simulink model "TAYCAN_MODEL"  (R2025b)
settings: Solver=ode23t  StartTime=0.0  StopTime=10000  RelTol=1e-3
values from neighbouring files (symbols this model uses):
  g = 9.81    [DRIVE_CYCLE_GEN.m]    (also in TAYCAN_PARAM_LOAD.m)
  L = 500    [TAYCAN_PARAM_LOAD.m]
  Max_brake_pressure_F_Bar = 200e5    (= 20000000)    [TAYCAN_PARAM_LOAD.m]
  Max_brake_pressure_R_Bar = 200e5    (= 20000000)    [TAYCAN_PARAM_LOAD.m]
  Max_torque_curve_F_Nm = Torque_x * Max_torque_curve_F_set    [Model_Sweeper.m]    (also in TAYCAN_PARAM_LOAD.m = [340;340;340;340;340;340;288.55;247.42;216.63;192.44;173.11;)
  Max_torque_curve_R_Nm = Torque_x * Max_torque_curve_R_set    [Model_Sweeper.m]    (also in TAYCAN_PARAM_LOAD.m = [900.00;900.00;900.00;900.00;900.00;900.00;900.00;898.90;785)
  Max_torque_generator_Nm = -350    [TAYCAN_PARAM_LOAD.m]
  Np = ceil(Ipack / Imax)    [Model_Sweeper.m]    (also in TAYCAN_PARAM_LOAD.m = 33)
  Ns = 198    [TAYCAN_PARAM_LOAD.m]
  regen_bias = 0.3    [TAYCAN_PARAM_LOAD.m]
  RPM_curve_RPM_F = (0:1000:RPM_max_RPM_F)'    [TAYCAN_PARAM_LOAD.m]
  RPM_curve_RPM_R = (0:1000:RPM_max_RPM_R)'    [TAYCAN_PARAM_LOAD.m]
  shift_down_v = shift_down_v_set(ids)    [Model_Sweeper.m]    (also in TAYCAN_PARAM_LOAD.m = 60)
  shift_up_v = shift_up_v_set(ids)    [Model_Sweeper.m]    (also in TAYCAN_PARAM_LOAD.m = 80)
  Tot_vehicle_mass_kg = Vehicle_mass_unladen_kg + Driver_mass_kg + batt_mass    [Model_Sweeper.m]    (also in TAYCAN_PARAM_LOAD.m = 2462.38)
  V_init = 4.2    [TAYCAN_PARAM_LOAD.m]
  VelDist = struct()    [DRIVE_CYCLE_GEN.m]    (also in VelocityVsDistance.mat = )
undefined symbols (not defined in the file or in its folder): Driver_Ki, Driver_Kp, Max_torque_motor_F__Nm, Max_torque_motor_R__Nm, Neg, Pos
libraries: fl_lib x23, nesl_utility x16, sdl_lib x15, batteryecm_lib x1, autolibshared x1
(part 1 of 2)
settings Model: Creator=User  LastModifiedBy=User

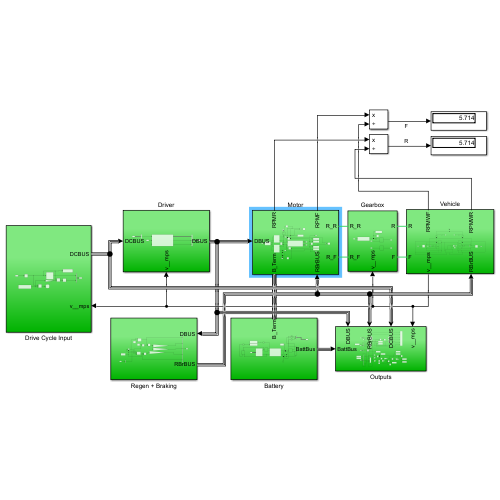
[thumbnail: Simulink's stored preview of the top-level diagram]
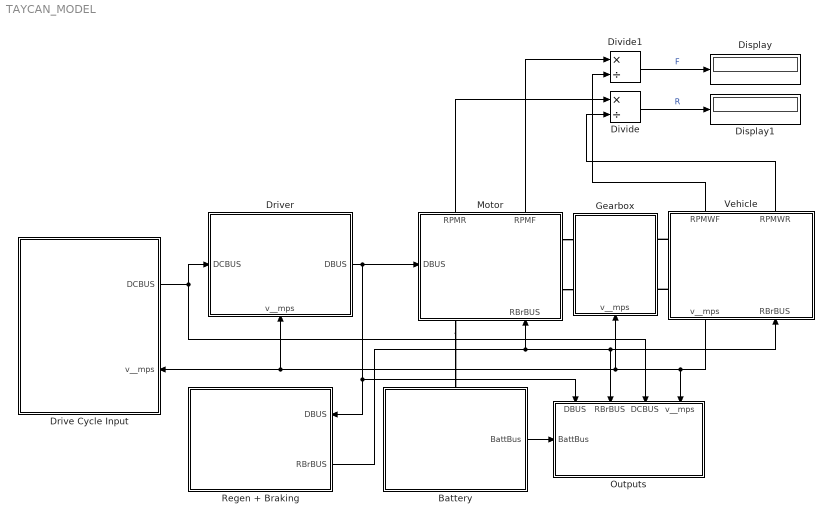
== system TAYCAN_MODEL ==
  Battery : Subsystem
      settings: PortSchema="{\"entries\":[{\"content\":{\"sides\":[{\"content\":{},\"type\":\"ConnectorPlacement.EquallySpacedRectSide\",\"uuid\":\"d14577cf-04a7-401a-8516-23c16a1412d1\"},{\"content\":{\"connectorIds\":[\"Out1\"],\"side\":\"RIGHT\"},\"type\":\"ConnectorPlacement.EquallySpacedRectSide\",\"uuid\":\"4e7522c9-8180-4e2e-bebe-28528e500786\"},{\"content\":{\"connectorIds\":[\"LConn1\"],\"side\":\"TOP\"},\"type\":\"ConnectorPlacement.EquallySpacedRectSide\",\"uuid\":\"3070fdfd-0295-4330-8a72-ca6da87c971c\"}]},\"type\":\"ConnectorPlacement.EquallySpacedConnector\",\"uuid\":\"084f7575-2e43-4328-abba-c452195d4f2d\"}],\"packageUris\":[\"http://schema.mathworks.com/mf0/Connector/R2020b\"],\"version\":\"1.0\"}"
  Display : Display
  Display1 : Display
  Divide : Product  Inputs=*/
  Divide1 : Product  Inputs=*/
  Drive Cycle Input : Subsystem
      settings: PortSchema="{\"entries\":[{\"content\":{\"sides\":[{\"content\":{},\"type\":\"ConnectorPlacement.EquallySpacedRectSide\",\"uuid\":\"0e92d9b4-4c78-4478-9d26-ea78bebdd29e\"},{\"content\":{\"connectorIds\":[\"Out1\",\"In1\"],\"side\":\"RIGHT\"},\"type\":\"ConnectorPlacement.EquallySpacedRectSide\",\"uuid\":\"045dcab9-f8e3-4899-a832-b3da2cc9584c\"},{\"content\":{\"side\":\"TOP\"},\"type\":\"ConnectorPlacement.EquallySpacedRectSide\",\"uuid\":\"84c167e0-eb64-4122-830b-befac4af6cd8\"}]},\"type\":\"ConnectorPlacement.EquallySpacedConnector\",\"uuid\":\"e4b995ab-b6cb-45a0-892e-35ade84b02de\"}],\"packageUris\":[\"http://schema.mathworks.com/mf0/Connector/R2020b\"],\"version\":\"1.0\"}"
  Driver : Subsystem
      settings: PortSchema="{\"entries\":[{\"content\":{\"sides\":[{\"content\":{\"connectorIds\":[\"In1\"]},\"type\":\"ConnectorPlacement.EquallySpacedRectSide\",\"uuid\":\"d14577cf-04a7-401a-8516-23c16a1412d1\"},{\"content\":{\"connectorIds\":[\"Out1\"],\"side\":\"RIGHT\"},\"type\":\"ConnectorPlacement.EquallySpacedRectSide\",\"uuid\":\"4e7522c9-8180-4e2e-bebe-28528e500786\"},{\"content\":{\"side\":\"TOP\"},\"type\":\"ConnectorPlacement.EquallySpacedRectSide\",\"uuid\":\"3070fdfd-0295-4330-8a72-ca6da87c971c\"},{\"content\":{\"connectorIds\":[\"In2\"],\"side\":\"BOTTOM\"},\"type\":\"ConnectorPlacement.EquallySpacedRectSide\",\"uuid\":\"fab3bc93-710b-429a-bed2-c063f5086687\"}]},\"type\":\"ConnectorPlacement.EquallySpacedConnector\",\"uuid\":\"084f7575-2e43-4328-abba-c452195d4f2d\"}],\"packageUris\":[\"http://schema.mathworks.com/mf0/Connector/R2020b\"],\"version\":\"1.0\"}"
  Gearbox : Subsystem
      settings: PortSchema="{\"entries\":[{\"content\":{\"sides\":[{\"content\":{\"connectorIds\":[\"LConn1\",\"LConn2\"]},\"type\":\"ConnectorPlacement.EquallySpacedRectSide\",\"uuid\":\"2cd79867-e1b6-4457-a4ee-a2c785994971\"},{\"content\":{\"connectorIds\":[\"RConn1\",\"RConn2\"],\"side\":\"RIGHT\"},\"type\":\"ConnectorPlacement.EquallySpacedRectSide\",\"uuid\":\"6eaf45d6-e5e8-4926-a6cd-7ecafda04af6\"},{\"content\":{\"side\":\"TOP\"},\"type\":\"ConnectorPlacement.EquallySpacedRectSide\",\"uuid\":\"07ebaeb6-dff9-4024-8855-2c554193f291\"},{\"content\":{\"connectorIds\":[\"In1\"],\"side\":\"BOTTOM\"},\"type\":\"ConnectorPlacement.EquallySpacedRectSide\",\"uuid\":\"50a107d2-832e-4284-8017-5113a03ebe7e\"}]},\"type\":\"ConnectorPlacement.EquallySpacedConnector\",\"uuid\":\"a35e96de-fd7f-4562-8d12-582ef1b75d5a\"}],\"packageUris\":[\"http://schema.mathworks.com/mf0/Connector/R2020b\"],\"version\":\"1.0\"}"
  Motor : Subsystem
      settings: PortSchema="{\"entries\":[{\"content\":{\"sides\":[{\"content\":{\"connectorIds\":[\"In1\"]},\"type\":\"ConnectorPlacement.EquallySpacedRectSide\",\"uuid\":\"4b804e5c-215d-420c-8cbc-4aec0c1bc9ed\"},{\"content\":{\"connectorIds\":[\"RConn1\",\"RConn2\"],\"side\":\"RIGHT\"},\"type\":\"ConnectorPlacement.EquallySpacedRectSide\",\"uuid\":\"7b3b7faa-3322-4a2b-ad45-f514a2b82e50\"},{\"content\":{\"connectorIds\":[\"Out1\",\"Out2\"],\"side\":\"TOP\"},\"type\":\"ConnectorPlacement.EquallySpacedRectSide\",\"uuid\":\"5f544e79-0644-465e-82e8-8009d644c481\"},{\"content\":{\"connectorIds\":[\"RConn3\",\"In2\"],\"side\":\"BOTTOM\"},\"type\":\"ConnectorPlacement.EquallySpacedRectSide\",\"uuid\":\"86807711-4ed8-4d7d-bac7-3eec1d423299\"}]},\"type\":\"ConnectorPlacement.EquallySpacedConnector\",\"uuid\":\"43c8d4a0-f993-46a1-82cf-86d7211b01ab\"}],\"packageUris\":[\"http://schema.mathworks.com/mf0/Connector/R2020b\"],\"version\":\"1.0\"}"
  Outputs : Subsystem
      settings: PortSchema="{\"entries\":[{\"content\":{\"sides\":[{\"content\":{\"connectorIds\":[\"In1\"]},\"type\":\"ConnectorPlacement.EquallySpacedRectSide\",\"uuid\":\"4d7fb8f9-77c0-425d-b0db-40d5e7c47a92\"},{\"content\":{\"side\":\"RIGHT\"},\"type\":\"ConnectorPlacement.EquallySpacedRectSide\",\"uuid\":\"49f936f9-7703-4fe0-b084-ec330908125c\"},{\"content\":{\"connectorIds\":[\"In2\",\"In3\",\"In4\",\"In5\"],\"side\":\"TOP\"},\"type\":\"ConnectorPlacement.EquallySpacedRectSide\",\"uuid\":\"def830fe-aace-4bb5-b5d5-c0664cb17e7e\"}]},\"type\":\"ConnectorPlacement.EquallySpacedConnector\",\"uuid\":\"0cef2ee5-170a-4149-8339-c8d04dee8bf4\"}],\"packageUris\":[\"http://schema.mathworks.com/mf0/Connector/R2020b\"],\"version\":\"1.0\"}"
  Regen + Braking : Subsystem
      settings: PortSchema="{\"entries\":[{\"content\":{\"sides\":[{\"content\":{},\"type\":\"ConnectorPlacement.EquallySpacedRectSide\",\"uuid\":\"79700970-756d-4ec6-8397-66d283bd30cc\"},{\"content\":{\"connectorIds\":[\"In1\",\"Out1\"],\"side\":\"RIGHT\"},\"type\":\"ConnectorPlacement.EquallySpacedRectSide\",\"uuid\":\"0add4294-302d-47bb-9f16-d681ae85b118\"},{\"content\":{\"side\":\"TOP\"},\"type\":\"ConnectorPlacement.EquallySpacedRectSide\",\"uuid\":\"37b62eba-8f15-40cb-afea-bce2353388c7\"}]},\"type\":\"ConnectorPlacement.EquallySpacedConnector\",\"uuid\":\"23d4a446-c033-44e5-854e-98cdd3b391c4\"}],\"packageUris\":[\"http://schema.mathworks.com/mf0/Connector/R2020b\"],\"version\":\"1.0\"}"
  Vehicle : Subsystem
      settings: PortSchema="{\"entries\":[{\"content\":{\"sides\":[{\"content\":{\"connectorIds\":[\"LConn1\",\"LConn2\"]},\"type\":\"ConnectorPlacement.EquallySpacedRectSide\",\"uuid\":\"2204119d-64df-494d-bdf6-dd5790b6a648\"},{\"content\":{\"side\":\"RIGHT\"},\"type\":\"ConnectorPlacement.EquallySpacedRectSide\",\"uuid\":\"957baec1-6ccf-49eb-9229-dff958c69421\"},{\"content\":{\"connectorIds\":[\"Out2\",\"Out3\"],\"side\":\"TOP\"},\"type\":\"ConnectorPlacement.EquallySpacedRectSide\",\"uuid\":\"91f4ac47-3518-4f09-ad19-4e7ac2e2af90\"},{\"content\":{\"connectorIds\":[\"Out1\",\"In1\"],\"side\":\"BOTTOM\"},\"type\":\"ConnectorPlacement.EquallySpacedRectSide\",\"uuid\":\"9fc835d4-3802-4793-8215-dc50523f1a5f\"}]},\"type\":\"ConnectorPlacement.EquallySpacedConnector\",\"uuid\":\"d2ba5914-f28e-4439-8569-04c9912b493f\"}],\"packageUris\":[\"http://schema.mathworks.com/mf0/Connector/R2020b\"],\"version\":\"1.0\"}"
  wires:
  Drive Cycle Input/1(DCBUS) -> Driver/1(DCBUS), Outputs/4(DCBUS)
  Vehicle/1(v__mps) -> Drive Cycle Input/1(v__mps), Driver/2(v__mps), Gearbox/1(v__mps), Outputs/5(v__mps)
  Driver/1(DBUS) -> Outputs/2(DBUS), Regen + Braking/1(DBUS), Motor/1(DBUS)
  Regen + Braking/1(RBrBUS) -> Vehicle/1(RBrBUS), Outputs/3(RBrBUS), Motor/2(RBrBUS)
  Battery/1(BattBus) -> Outputs/1(BattBus)
  Motor/1(RPMR) -> Divide/1
  Vehicle/3(RPMWR) -> Divide/2
  Vehicle/2(RPMWF) -> Divide1/2
  Motor/2(RPMF) -> Divide1/1
  Divide1/1 -> Display/1  "F"
  Divide/1 -> Display1/1  "R"
  connections:
  Motor/RConn3 -- Battery/LConn1
  Motor/RConn1 -- Gearbox/LConn1
  Motor/RConn2 -- Gearbox/LConn2
  Vehicle/LConn1 -- Gearbox/RConn1
  Vehicle/LConn2 -- Gearbox/RConn2

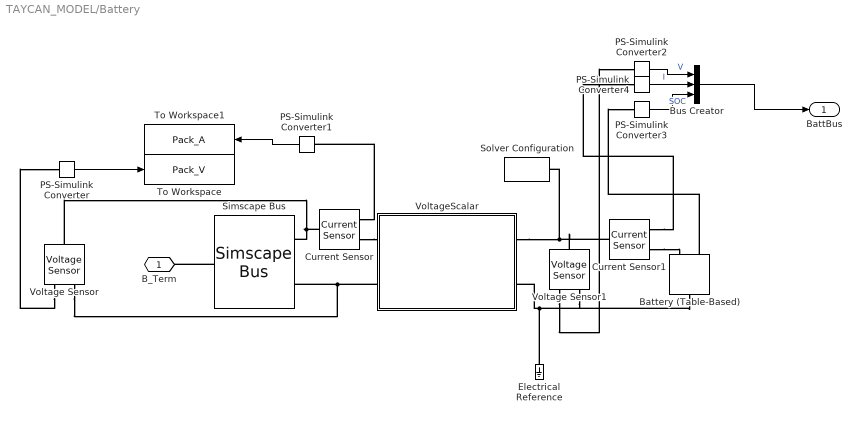
== system TAYCAN_MODEL/Battery ==
  Battery (Table-Based) : batteryecm_lib/Battery (Table-Based)  PartSpecification="{\"CollectionId\":\"SimscapeBatteryShared\",\"CollectionVersion\":\"1.0.0\",\"DatasetId\":\"Molicel|INR_21700_P45B|simscape.battery.batteryTableBased\",\"DisplayName\":\"Molicel:INR_21700_P45B\"}"  SOC_vec=[0 0.01 0.02 0.03 0.04 0.05 0.06 0.07 0.08 0.09 0.1 0.11 0.12 0.13 0.14 0.15 0.16 0.17 0.18 0.19 0.2 0.21 0.22 0.23 0.24 0.25 0.26 0.27 0.28 0.29 0.3 0.31 0.32 0.33 0.34 0.35 0.36 0.37 0.38 0.39 0.4 0.41 0.42 0.43 0.44 0.45 0.46 0.47 0.48 0.49 0.5 0.51 0.52 0.53 0.54 0.55 0.56 0.57 0.58 0.59 0.6 0.61 0.62 0.63 0.64 0.65 0.66 0.67 0.68 0.69 0.7 0.71 0.72 0.73 0.74 0.75 0.76 0.77 0.78 0.79 0.8 0.81 0.82 0.83 0.84 0.85 0.86 0.87 0.88 0.89 0.9 0.91 0.92 0.93 0.94 0.95 0.96 0.97 0.98 0.99 1] % Datasheet derived  T_dependence=simscape.enum.tablebattery.temperature_dependence.yes  prm_dir=simscape.enum.tablebattery.prm_dir.noCurrentDirectionality  T_vec=[-40 -30 -20 0 23 45 60] % Datasheet derived degC  V0_mat=[3.17242 3.17242 3.17242 3.17242 3.17242 3.17242 3.17242;3.18272 3.18272 3.18272 3.18272 3.18272 3.18272 3.18272;3.19302 3.19302 3.19302 3.19302 3.19302 3.19302 3.19302;3.20331 3.20331 3.20331 3.20331 3.20331 3.20331 3.20331;3.21361 3.21361 3.21361 3.21361 3.21361 3.21361 3.21361;3.22391 3.22391 3.22391 3.22391 3.22391 3.22391 3.22391;3.23421 3.23421 3.23421 3.23421 3.23421 3.23421 3.23421;3.24451 3.24451 3.24451 3.24451 3.24451 3.24451 3.24451;3.25481 3.25481 3.25481 3.25481 3.25481 3.25481 3.25481;3.2651 3.2651 3.2651 3.2651 3.2651 3.2651 3.2651;3.2754 3.2754 3.2754 3.2754 3.2754 3.2754 3.2754;3.2857 3.2857 3.2857 3.2857 3.2857 3.2857 3.2857;3.296 3.296 3.296 3.296 3.296 3.296 3.296;3.3063 3.3063 3.3063 3.3063 3.3063 3.3063 3.3063;3.31659 3.31659 3.31659 3.31659 3.31659 3.31659 3.31659;3.32689 3.32689 3.32689 3.32689 3.32689 3.32689 3.32689;3.33719 3.33719 3.33719 3.33719 3.33719 3.33719 3.33719;3.34749 3.34749 3.34749 3.34749 3.34749 3.34749 3.34749;3.35779 3.35779 3.35779 3.35779 3.35779 3.35779 3.35779;3.36809 3.36809 3.36809 3.36809 3.36809 3.36809 3.36809;3.37838 3.37838 3.37838 3.37838 3.37838 3.37838 3.37838;3.38868 3.38868 3.38868 3.38868 3.38868 3.38868 3.38868;3.39898 3.39898 3.39898 3.39898 3.39898 3.39898 3.39898;3.40928 3.40928 3.40928 3.40928 3.40928 3.40928 3.40928;3.41958 3.41958 3.41958 3.41958 3.41958 3.41958 3.41958;3.42988 3.42988 3.42988 3.42988 3.42988 3.42988 3.42988;3.44017 3.44017 3.44017 3.44017 3.44017 3.44017 3.44017;3.45047 3.45047 3.45047 3.45047 3.45047 3.45047 3.45047;3.46077 3.46077 3.46077 3.46077 3.46077 3.46077 3.46077;3.47107 3.47107 3.47107 3.47107 3.47107 3.47107 3.47107;3.48137 3.48137 3.48137 3.48137 3.48137 3.48137 3.48137;3.49166 3.49166 3.49166 3.49166 3.49166 3.49166 3.49166;3.50196 3.50196 3.50196 3.50196 3.50196 3.50196 3.50196;3.51226 3.51226 3.51226 3.51226 3.51226 3.51226 3.51226;3.52256 3.52256 3.52256 3.52256 3.52256 3.52256 3.52256;3.53286 3.53286 3.53286 3.53286 3.53286 3.53286 3.53286;3.54316 3.54316 3.54316 3.54316 3.54316 3.54316 3.54316;3.55345 3.55345 3.55345 3.55345 3.55345 3.55345 3.55345;3.56375 3.56375 3.56375 3.56375 3.56375 3.56375 3.56375;3.57405 3.57405 3.57405 3.57405 3.57405 3.57405 3.57405;3.58435 3.58435 3.58435 3.58435 3.58435 3.58435 3.58435;3.59465 3.59465 3.59465 3.59465 3.59465 3.59465 3.59465;3.60495 3.60495 3.60495 3.60495 3.60495 3.60495 3.60495;3.61524 3.61524 3.61524 3.61524 3.61524 3.61524 3.61524;3.62554 3.62554 3.62554 3.62554 3.62554 3.62554 3.62554;3.63584 3.63584 3.63584 3.63584 3.63584 3.63584 3.63584;3.64614 3.64614 3.64614 3.64614 3.64614 3.64614 3.64614;3.65644 3.65644 3.65644 3.65644 3.65644 3.65644 3.65644;3.66673 3.66673 3.66673 3.66673 3.66673 3.66673 3.66673;3.67703 3.67703 3.67703 3.67703 3.67703 3.67703 3.67703;3.68733 3.68733 3.68733 3.68733 3.68733 3.68733 3.68733;3.69763 3.69763 3.69763 3.69763 3.69763 3.69763 3.69763;3.71041 3.71041 3.71041 3.71041 3.71041 3.71041 3.71041;3.72113 3.72113 3.72113 3.72113 3.72113 3.72113 3.72113;3.72997 3.72997 3.72997 3.72997 3.72997 3.72997 3.72997;3.73882 3.73882 3.73882 3.73882 3.73882 3.73882 3.73882;3.74912 3.74912 3.74912 3.74912 3.74912 3.74912 3.74912;3.75936 3.75936 3.75936 3.75936 3.75936 3.75936 3.75936;3.76951 3.76951 3.76951 3.76951 3.76951 3.76951 3.76951;3.7791 3.7791 3.7791 3.7791 3.7791 3.7791 3.7791;3.78865 3.78865 3.78865 3.78865 3.78865 3.78865 3.78865;3.79787 3.79787 3.79787 3.79787 3.79787 3.79787 3.79787;3.80709 3.80709 3.80709 3.80709 3.80709 3.80709 3.80709;3.8161 3.8161 3.8161 3.8161 3.8161 3.8161 3.8161;3.82509 3.82509 3.82509 3.82509 3.82509 3.82509 3.82509;3.83409 3.83409 3.83409 3.83409 3.83409 3.83409 3.83409;3.84308 3.84308 3.84308 3.84308 3.84308 3.84308 3.84308;3.85207 3.85207 3.85207 3.85207 3.85207 3.85207 3.85207;3.86107 3.86107 3.86107 3.86107 3.86107 3.86107 3.86107;3.87006 3.87006 3.87006 3.87006 3.87006 3.87006 3.87006;3.87901 3.87901 3.87901 3.87901 3.87901 3.87901 3.87901;3.88831 3.88831 3.88831 3.88831 3.88831 3.88831 3.88831;3.89824 3.89824 ...(+1594 chars)] % Datasheet derived V  V0_vec=[3.17242 3.18272 3.19302 3.20331 3.21361 3.22391 3.23421 3.24451 3.25481 3.2651 3.2754 3.2857 3.296 3.3063 3.31659 3.32689 3.33719 3.34749 3.35779 3.36809 3.37838 3.38868 3.39898 3.40928 3.41958 3.42988 3.44017 3.45047 3.46077 3.47107 3.48137 3.49166 3.50196 3.51226 3.52256 3.53286 3.54316 3.55345 3.56375 3.57405 3.58435 3.59465 3.60495 3.61524 3.62554 3.63584 3.64614 3.65644 3.66673 3.67703 3.68733 3.69763 3.71041 3.72113 3.72997 3.73882 3.74912 3.75936 3.76951 3.7791 3.78865 3.79787 3.80709 3.8161 3.82509 3.83409 3.84308 3.85207 3.86107 3.87006 3.87901 3.88831 3.89824 3.90887 3.91951 3.93012 3.94073 3.95138 3.96184 3.97226 3.98268 3.99311 4.0032 4.01221 4.01944 4.02668 4.03286 4.03874 4.04383 4.0488 4.05377 4.05873 4.06312 4.06753 4.07333 4.08117 4.08904 4.09911 4.11111 4.13802 4.16831] % Datasheet derived V  V_range=[2.25 Inf] % Datasheet derived V  R0_mat=[0.3026 0.35142 0.34349 0.24415 0.02095 0.15874 0.14729;0.2941 0.33555 0.32379 0.22614 0.01921 0.13363 0.12249;0.28559 0.31969 0.30408 0.20813 0.01774 0.10853 0.10276;0.27709 0.30382 0.28438 0.19012 0.0166 0.09423 0.0861;0.26858 0.28796 0.26468 0.17211 0.01557 0.07998 0.0748;0.26008 0.27209 0.24498 0.1541 0.01469 0.07024 0.06679;0.25157 0.25623 0.22527 0.1361 0.01398 0.06387 0.05877;0.24307 0.24036 0.20557 0.11861 0.01338 0.0575 0.05275;0.23456 0.2245 0.18587 0.10674 0.01283 0.05113 0.04899;0.22606 0.20863 0.16617 0.09525 0.01239 0.04679 0.04522;0.21755 0.19277 0.14651 0.08799 0.01196 0.0439 0.04145;0.20905 0.1769 0.13098 0.08073 0.01155 0.04101 0.03817;0.20054 0.16103 0.11905 0.07347 0.01116 0.03813 0.03522;0.19204 0.14769 0.11102 0.06895 0.01079 0.03524 0.03228;0.18353 0.13913 0.10517 0.06499 0.01042 0.03235 0.02934;0.17503 0.13157 0.09933 0.06104 0.01007 0.02946 0.0264;0.16653 0.1271 0.09371 0.05708 0.00974 0.02657 0.02345;0.15804 0.12264 0.09094 0.05312 0.00949 0.02417 0.02125;0.15354 0.11817 0.08816 0.04917 0.00924 0.02286 0.01972;0.14976 0.11385 0.08539 0.04748 0.009 0.02156 0.0182;0.14598 0.11213 0.08261 0.04617 0.00876 0.02025 0.01667;0.14219 0.11042 0.08103 0.04487 0.00855 0.01894 0.01515;0.14033 0.10871 0.08035 0.04356 0.00843 0.01763 0.01363;0.13876 0.10699 0.07967 0.04225 0.00832 0.01632 0.0121;0.13718 0.10528 0.07899 0.04094 0.00826 0.01501 0.01058;0.13561 0.10357 0.07831 0.03964 0.00825 0.0137 0.00906;0.13404 0.10198 0.07763 0.03833 0.00825 0.01239 0.00753;0.13247 0.10119 0.07695 0.03702 0.00826 0.01108 0.0065;0.13096 0.10039 0.07627 0.03624 0.00827 0.00977 0.00633;0.13043 0.0996 0.07559 0.03615 0.00828 0.00846 0.00617;0.1299 0.0988 0.07491 0.03606 0.0083 0.00774 0.006;0.12937 0.09801 0.07423 0.03597 0.00834 0.00779 0.00583;0.12883 0.09721 0.07355 0.03588 0.00838 0.00783 0.00567;0.1283 0.09642 0.07301 0.03579 0.00842 0.00787 0.0055;0.12777 0.09585 0.07296 0.0357 0.00848 0.00792 0.00534;0.12724 0.09584 0.07291 0.03561 0.00855 0.00796 0.00517;0.12675 0.09584 0.07286 0.03552 0.00863 0.00801 0.005;0.12643 0.09583 0.0728 0.03543 0.00871 0.00805 0.00484;0.12611 0.09582 0.07275 0.03534 0.00879 0.00809 0.00467;0.12579 0.09582 0.0727 0.03525 0.00887 0.00814 0.0045;0.12547 0.09581 0.07264 0.03526 0.00895 0.00818 0.00434;0.12514 0.0958 0.07259 0.03537 0.00903 0.00823 0.00405;0.12482 0.09579 0.07254 0.03547 0.00911 0.00804 0.00366;0.1245 0.09579 0.07248 0.03558 0.00918 0.00776 0.00327;0.12418 0.09578 0.07243 0.03568 0.00925 0.00748 0.00287;0.12386 0.09577 0.07231 0.03579 0.00931 0.0072 0.00248;0.12354 0.09576 0.0721 0.03589 0.00938 0.00692 0.00209;0.12322 0.09576 0.07189 0.036 0.00946 0.00664 0.0017;0.12301 0.09575 0.07168 0.03611 0.00953 0.00636 0.00131;0.12309 0.09574 0.07147 0.03621 0.00961 0.00608 0.00092;0.12318 0.09573 0.07125 0.0363 0.00968 0.0058 0.00053;0.12326 0.09573 0.07104 0.03637 0.00976 0.00552 0.00014;0.12389 0.09628 0.07138 0.03699 0.00991 0.00579 0.0003;0.12407 0.09637 0.07126 0.03715 0.01 0.0056 0.0003;0.12383 0.09605 0.07073 0.0369 0.01003 0.00504 0.0003;0.12359 0.09573 0.07019 0.03664 0.01006 0.00503 0.0003;0.12367 0.09573 0.06998 0.03671 0.01013 0.00534 0.00063;0.12375 0.09572 0.06975 0.03677 0.01022 0.00564 0.00094;0.1238 0.09569 0.07006 0.0368 0.0103 0.00593 0.00123;0.12372 0.09554 0.07026 0.03671 0.01037 0.00608 0.00139;0.12364 0.09537 0.07046 0.03661 0.01043 0.00623 0.00155;0.12348 0.09514 0.07058 0.03644 0.01049 0.0063 0.00163;0.12333 0.0949 0.07071 0.03627 0.01055 0.00638 0.00171;0.12312 0.09461 0.07078 0.03605 0.01061 0.00641 0.00175;0.12291 0.09433 0.07085 0.03583 0.01066 0.00643 0.00168;0.12271 0.09404 0.07093 0.03568 0.01072 0.00646 0.00161;0.12275 0.09398 0.071 0.03622 0.01077 0.00646 0.00153;0.12316 0.09449 0.07107 0.03677 0.01082 0.00636 0.00145;0.12357 0.095 0.07115 0.03731 0.01088 0.00625 0.00137;0.12398 0.09551 0.07151 0.03785 0.01093 0.00614 0.00129;0.12438 0.09601 0.07221 0.03839 0.01099 0.00602 0.0012;0.12486 0.09659 0.07299 0.039 0.01105 0.00599 0.00119;0.12548 0.09731 0.07391 ...(+1579 chars)] % Datasheet derived Ohm  R0_vec=[0.02095 0.01921 0.01774 0.0166 0.01557 0.01469 0.01398 0.01338 0.01283 0.01239 0.01196 0.01155 0.01116 0.01079 0.01042 0.01007 0.00974 0.00949 0.00924 0.009 0.00876 0.00855 0.00843 0.00832 0.00826 0.00825 0.00825 0.00826 0.00827 0.00828 0.0083 0.00834 0.00838 0.00842 0.00848 0.00855 0.00863 0.00871 0.00879 0.00887 0.00895 0.00903 0.00911 0.00918 0.00925 0.00931 0.00938 0.00946 0.00953 0.00961 0.00968 0.00976 0.00991 0.01 0.01003 0.01006 0.01013 0.01022 0.0103 0.01037 0.01043 0.01049 0.01055 0.01061 0.01066 0.01072 0.01077 0.01082 0.01088 0.01093 0.01099 0.01105 0.01114 0.01125 0.01136 0.01148 0.01161 0.01175 0.01188 0.01202 0.01215 0.01228 0.01241 0.01253 0.01261 0.01269 0.01275 0.0128 0.01285 0.01289 0.01294 0.01298 0.01296 0.01292 0.01292 0.01288 0.01282 0.0128 0.01232 0.01214 0.00952] % Datasheet derived Ohm  R0_dis_mat=[.0117, .0085, .009; .011, .0085, .009; .0114, .0087, .0092; .0107, .0082, .0088; .0107, .0083, .0091; .0113, .0085, .0089; .0116, .0085, .0089] % Parameter not set Ohm  R0_dis_vec=[.0085, .0085, .0087, .0082, .0083, .0085, .0085] % Parameter not set Ohm  R0_ch_mat=[.0117, .0085, .009; .011, .0085, .009; .0114, .0087, .0092; .0107, .0082, .0088; .0107, .0083, .0091; .0113, .0085, .0089; .0116, .0085, .0089] % Parameter not set Ohm  R0_ch_vec=[.0085, .0085, .0087, .0082, .0083, .0085, .0085] % Parameter not set Ohm  AH=4.493 % Datasheet derived hr*A  prm_leak=simscape.enum.tablebattery.prm_leak.disabled  Rleak_vec=[8000, 7000, 6000] % Parameter not set Ohm  Rleak=7e3 % Parameter not set Ohm  extrapolation_option=simscape.enum.extrapolation.nearest  SOC_port=simscape.enum.tablebattery.enable.yes  prm_dyn=simscape.enum.tablebattery.prm_dyn.off  R1_mat=[.0109, .0029, .0013; .0069, .0024, .0012; .0047, .0026, .0013; .0034, .0016, .001; .0033, .0023, .0014; .0033, .0018, .0011; .0028, .0017, .0011] % Parameter not set Ohm  R1_vec=[.0029, .0024, .0026, .0016, .0023, .0018, .0017] % Parameter not set Ohm  tau1_mat=[20, 36, 39; 31, 45, 39; 109, 105, 61; 36, 29, 26; 59, 77, 67; 40, 33, 29; 25, 39, 33] % Parameter not set s  tau1_vec=[36, 45, 105, 29, 77, 33, 39] % Parameter not set s  R2_mat=[.0109, .0029, .0013; .0069, .0024, .0012; .0047, .0026, .0013; .0034, .0016, .001; .0033, .0023, .0014; .0033, .0018, .0011; .0028, .0017, .0011] % Parameter not set Ohm  R2_vec=[.0029, .0024, .0026, .0016, .0023, .0018, .0017] % Parameter not set Ohm  tau2_mat=[20, 36, 39; 31, 45, 39; 109, 105, 61; 36, 29, 26; 59, 77, 67; 40, 33, 29; 25, 39, 33] % Parameter not set s  tau2_vec=[36, 45, 105, 29, 77, 33, 39] % Parameter not set s  R3_mat=[.0109, .0029, .0013; .0069, .0024, .0012; .0047, .0026, .0013; .0034, .0016, .001; .0033, .0023, .0014; .0033, .0018, .0011; .0028, .0017, .0011] % Parameter not set Ohm  R3_vec=[.0029, .0024, .0026, .0016, .0023, .0018, .0017] % Parameter not set Ohm  tau3_mat=[20, 36, 39; 31, 45, 39; 109, 105, 61; 36, 29, 26; 59, 77, 67; 40, 33, 29; 25, 39, 33] % Parameter not set s  tau3_vec=[36, 45, 105, 29, 77, 33, 39] % Parameter not set s  R4_mat=[.0109, .0029, .0013; .0069, .0024, .0012; .0047, .0026, .0013; .0034, .0016, .001; .0033, .0023, .0014; .0033, .0018, .0011; .0028, .0017, .0011] % Parameter not set Ohm  R4_vec=[.0029, .0024, .0026, .0016, .0023, .0018, .0017] % Parameter not set Ohm  tau4_mat=[20, 36, 39; 31, 45, 39; 109, 105, 61; 36, 29, 26; 59, 77, 67; 40, 33, 29; 25, 39, 33] % Parameter not set s  tau4_vec=[36, 45, 105, 29, 77, 33, 39] % Parameter not set s  R5_mat=[.0109, .0029, .0013; .0069, .0024, .0012; .0047, .0026, .0013; .0034, .0016, .001; .0033, .0023, .0014; .0033, .0018, .0011; .0028, .0017, .0011] % Parameter not set Ohm  R5_vec=[.0029, .0024, .0026, .0016, .0023, .0018, .0017] % Parameter not set Ohm  tau5_mat=[20, 36, 39; 31, 45, 39; 109, 105, 61; 36, 29, 26; 59, 77, 67; 40, 33, 29; 25, 39, 33] % Parameter not set s  tau5_vec=[36, 45, 105, 29, 77, 33, 39] % Parameter not set s  prm_fade=simscape.enum.tablebattery.prm_fade.tableN  N0=100 % Parameter not set  dV0=0 % Parameter not set  dR0=0 % Parameter not set  dAH=0 % Parameter not set  dRleak=0 % Parameter not set  dR1=0 % Parameter not set  dR2=0 % Parameter not set  dR3=0 % Parameter not set  dR4=0 % Parameter not set  dR5=0 % Parameter not set  N0vec=[0 6 11 16 21 26 31 36 41 46 51 56 61 66 71 76 81 86 91 96 101 106 111 116 121 126 131 136 141 146 151 156 161 166 171 176 181 186 191 196 201 206 211 216 221 226 231 236 241 246 251 256 261 266 271 276 281 286 291 296 301 306 311 316 321 326 331 336 341 346 351 356 361 366 371 376 381 386 391 396 401 406 411 416 421 426 431 436 441 446 451 456 461 466 471 476 481 486 491 496] % Datasheet derived  Tfadevec=[298.15, 323.15] % Parameter not set K  dV0vec=[0 -0.0674 -0.1349 -0.2023 -0.2697 -0.3371 -0.4046 -0.472 -0.5394 -0.6069 -0.6828 -0.7561 -0.8245 -0.8929 -0.9613 -1.0297 -1.0981 -1.1664 -1.2348 -1.3032 -1.3773 -1.4186 -1.4598 -1.5011 -1.5424 -1.5836 -1.6249 -1.6652 -1.6999 -1.7345 -1.7691 -1.8038 -1.8384 -1.8731 -1.908 -1.9398 -1.9715 -2.0033 -2.0351 -2.0669 -2.0986 -2.1303 -2.162 -2.1976 -2.2332 -2.2687 -2.2977 -2.3239 -2.3502 -2.3765 -2.4028 -2.4264 -2.4464 -2.4663 -2.4863 -2.5063 -2.5263 -2.5462 -2.5661 -2.5849 -2.6031 -2.6212 -2.6407 -2.6612 -2.6817 -2.7022 -2.7227 -2.7432 -2.7637 -2.7842 -2.8047 -2.8253 -2.8458 -2.8662 -2.8858 -2.9054 -2.9249 -2.9445 -2.9641 -2.9837 -3.0037 -3.0238 -3.0439 -3.064 -3.0841 -3.1042 -3.1267 -3.1499 -3.1731 -3.1989 -3.2248 -3.2508 -3.2781 -3.3053 -3.3326 -3.3598 -3.387 -3.4171 -3.449 -3.4809] % Datasheet derived  dR0vec=[0 0 0 0 0 0 0 0 0 0 0 0 0 0 0 0 0 0 0 0 0 0 0 0 0 0 0 0 0 0 0 0 0 0 0 0 0 0 0 0 0 0 0 0 0 0 0 0 0 0 0 0 0 0 0 0 0 0 0 0 0 0 0 0 0 0 0 0 0 0 0 0 0 0 0 0 0 0 0 0 0 0 0 0 0 0 0 0 0 0 0 0 0 0 0 0 0 0 0 0] % Parameter assumed  dAHvec=[0 -0.093 -0.186 -0.278 -0.371 -0.464 -0.557 -0.649 -0.742 -0.835 -0.94 -1.045 -1.151 -1.257 -1.363 -1.469 -1.575 -1.681 -1.787 -1.893 -2.017 -2.161 -2.304 -2.447 -2.591 -2.734 -2.877 -3.021 -3.164 -3.307 -3.451 -3.594 -3.737 -3.881 -4.032 -4.201 -4.369 -4.538 -4.706 -4.874 -5.043 -5.211 -5.38 -5.569 -5.758 -5.947 -6.135 -6.324 -6.513 -6.702 -6.891 -7.08 -7.269 -7.458 -7.647 -7.836 -8.025 -8.214 -8.403 -8.582 -8.754 -8.927 -9.099 -9.271 -9.443 -9.615 -9.787 -9.96 -10.132 -10.304 -10.476 -10.648 -10.82 -10.992 -11.156 -11.32 -11.485 -11.649 -11.814 -11.978 -12.143 -12.307 -12.471 -12.636 -12.8 -12.965 -13.129 -13.293 -13.458 -13.641 -13.825 -14.008 -14.192 -14.376 -14.56 -14.743 -14.927 -15.111 -15.295 -15.478] % Datasheet derived  dRleakvec=[0, 0, 0, 0] % Parameter not set  dR1vec=[0, 0, 0, 0] % Parameter not set  dR2vec=[0, 0, 0, 0] % Parameter not set  dR3vec=[0, 0, 0, 0] % Parameter not set  dR4vec=[0, 0, 0, 0] % Parameter not set  dR5vec=[0, 0, 0, 0] % Parameter not set  dV0mat=[0, 0; 0, 0; 0, 0; 0, 0] % Parameter not set  dR0mat=[0, 0; 0, 0; 0, 0; 0, 0] % Parameter not set  dAHmat=[0, 0; 0, 0; 0, 0; 0, 0] % Parameter not set  dRleakmat=[0, 0; 0, 0; 0, 0; 0, 0] % Parameter not set  dR1mat=[0, 0; 0, 0; 0, 0; 0, 0] % Parameter not set  dR2mat=[0, 0; 0, 0; 0, 0; 0, 0] % Parameter not set  dR3mat=[0, 0; 0, 0; 0, 0; 0, 0] % Parameter not set  dR4mat=[0, 0; 0, 0; 0, 0; 0, 0] % Parameter not set  dR5mat=[0, 0; 0, 0; 0, 0; 0, 0] % Parameter not set  prm_age_modeling=simscape.enum.tablebattery.prm_age_modeling.equation  storage_dt_age_vec=[0] % Parameter not set d  storage_T_age_vec=[273] % Parameter not set K  prm_age_OCV=simscape.enum.tablebattery.prm_age_OCV.OCV  OCV_age=0.9 % Parameter not set  SOC_age=0.6 % Parameter not set  prm_age_resistance=simscape.enum.tablebattery.prm_age.disabled  OCV_scaling_age_resistance=2.2134e6 % Parameter not set  OCV_offset_age_resistance=1.632e6 % Parameter not set  temp_exp_age_resistance=0.515833569 % Parameter not set V  t_exp_age_resistance=0.75 % Parameter not set  T_age_vec_resistance=[273.15, 298.15, 323.15] % Parameter not set K  dt_age_vec_resistance=[0, 90, 180, 270] % Parameter not set d  dR0_age_vec=[0, 0, 0] % Parameter not set  t_meas_dR0_age=100 % Parameter not set d  dR0_age_mat=[0, 0, 0; 0, 0, 0; 0, 0, 0; 0, 0, 0] % Parameter not set  prm_age_capacity=simscape.enum.tablebattery.prm_age.disabled  OCV_scaling_age_capacity=1.5097e07 % Parameter not set  OCV_offset_age_capacity=8.3625e06 % Parameter not set  temp_exp_age_capacity=0.6011 % Parameter not set V  t_exp_age_capacity=0.75 % Parameter not set  T_age_vec_capacity=[273.15, 298.15, 323.15] % Parameter not set K  dt_age_vec_capacity=[0, 90, 180, 270] % Parameter not set d  dAH_age_vec=[0, 0, 0] % Parameter not set  t_meas_dAH_age=100 % Parameter not set d  dAH_age_mat=[0, 0, 0; 0, 0, 0; 0, 0, 0; 0, 0, 0] % Parameter not set  thermal_port=simscape.enum.thermaleffects.omit  temperature=298.15 % Parameter not set K  thermal_mass=63 % Parameter assumed J/K  i_specify=off  i_priority=None  i=0 A  i_nominal_specify=off  i_nominal_value=1  i_nominal_unit=A  v_specify=off  v_priority=None  v=0 V  v_nominal_specify=off  v_nominal_value=1  v_nominal_unit=V  stateOfCharge_specify=off  stateOfCharge_priority=High  stateOfCharge=1  stateOfCharge_nominal_specify=off  stateOfCharge_nominal_value=1  stateOfCharge_nominal_unit=1  num_cycles_specify=off  num_cycles_priority=High  num_cycles=0  num_cycles_nominal_specify=off  num_cycles_nominal_value=1  num_cycles_nominal_unit=1  cell_temperature_specify=off  cell_temperature_priority=High  cell_temperature=298.15 K  cell_temperature_nominal_specify=off  cell_temperature_nominal_value=1  cell_temperature_nominal_unit=K
      settings: AttributesFormatString=Molicel:INR_21700_P45B  InternalSimscapePortConfiguration="{\"Bottom\":[],\"Left\":[{\"id\":\"p\",\"label\":\"+\",\"type\":\"foundation.electrical.electrical\"},{\"id\":\"soc\",\"label\":\"SOC\",\"type\":\"output\"}],\"Right\":[{\"id\":\"n\",\"label\":\"-\",\"type\":\"foundation.electrical.electrical\"}],\"Top\":[]}"
      settings: LibrarySourceBlock=|
      | batt_lib/Cells/Battery
      | (Table-Based)
  Bus Creator : BusCreator  Inputs=3
  Current Sensor : fl_lib/Electrical/Electrical Sensors/Current Sensor
  Current Sensor1 : fl_lib/Electrical/Electrical Sensors/Current Sensor
  Electrical Reference : fl_lib/Electrical/Electrical Elements/Electrical Reference
  PS-Simulink Converter{,1..4} (5 alike) : nesl_utility/PS-Simulink Converter  PhysicalDomain=network_engine_domain  SubClassName=ps_output  LeftPortType=input  RightPortType=output  PseudoPeriodic=off  Frequencies=[]  VectorFormat=inherit  Unit=inherit  AffineConversion=off
  Simscape Bus : SimscapeBus  HierarchyStrings=Pos;Neg
  Solver Configuration : nesl_utility/Solver Configuration  PhysicalDomain=network_engine_domain  SubClassName=solver  LeftPortType=input  RightPortType=generic  Tones=[]  Harmonics=[]  SimulateNoise=off  Profile=off  UseLocalSampling=off  EnableSwitchedLinearOptims=on  FrequencyDomain=off  UseCCode=off  RelTol=0.001  AbsTol=1e-06  MinStep=1e-09  ToWorkspace=off  RevertToSquareIcSolve=off  NumHomotopyIterations=100  PhasorMode=off  PhasorModeNumHarmonics=1  ConsistencySolver=NEWTON_XTOL_AFTER_FTOL  IndexReductionMethod=DerivativeReplacement  DoDC=off  ResidualTolerance=1e-9  ConsistencyTolSource=GLOBAL  ConsistencyAbsTol=0.001  ConsistencyRelTol=0.001  ConsistencyTolFactor=0.001  UseLocalSolver=on  LocalSolverChoice=NE_BACKWARD_EULER_ADVANCER  ResolveIndetEquations=on  FunctionEvalNumThread=1  LocalSolverSampleTime=0.001  DoFixedCost=off  MaxNonlinIter=3  MaxModeIter=2  ComputeImpulses=off  ImpulseIterations=2  LinearAlgebra=auto  LinearAlgebraNumThread=0  EquationFormulation=NE_TIME_EF  DelaysMemoryBudget=1024  AutomaticFiltering=on  FilteringTimeConstant=0.001  PartitionStorageMethod=AS_NEEDED  PartitionMemoryBudget=1024  PartitionMethod=FAST  MultibodyUseLocalSolver=off  MultibodyLocalSolverChoice=ODE1  MultibodyLocalSolverSampleTime=0.001
  To Workspace : ToWorkspace  VariableName=Pack_V  SaveFormat=Timeseries  SampleTime=-1
  To Workspace1 : ToWorkspace  VariableName=Pack_A  SaveFormat=Timeseries  SampleTime=-1
  Voltage Sensor : fl_lib/Electrical/Electrical Sensors/Voltage Sensor
  Voltage Sensor1 : fl_lib/Electrical/Electrical Sensors/Voltage Sensor
  VoltageScalar : Subsystem  mask{n_ser=Ns, n_para=Np, V_init=V_init, t_filt=0.001}
      mask prompts: V_init "V_init (unit)"
  B_Term : PMIOPort  Side=Left
  BattBus : Outport
  wires:
  Bus Creator/1 -> BattBus/1
  PS-Simulink Converter/1 -> To Workspace/1
  PS-Simulink Converter1/1 -> To Workspace1/1
  PS-Simulink Converter2/1 -> Bus Creator/1  "V"
  PS-Simulink Converter4/1 -> Bus Creator/2  "I"
  PS-Simulink Converter3/1 -> Bus Creator/3  "SOC"
  connections:
  Simscape Bus/RConn1 -- B_Term/RConn1
  VoltageScalar/LConn2 -- Voltage Sensor/RConn2 -- Simscape Bus/LConn2
  VoltageScalar/RConn1 -- Current Sensor1/LConn1 -- Voltage Sensor1/LConn1 -- Solver Configuration/RConn1
  Electrical Reference/LConn1 -- VoltageScalar/RConn2 -- Battery (Table-Based)/RConn1 -- Voltage Sensor1/RConn2
  Voltage Sensor/LConn1 -- Current Sensor/LConn1 -- Simscape Bus/LConn1
  Voltage Sensor/RConn1 -- PS-Simulink Converter/LConn1
  Current Sensor/RConn2 -- VoltageScalar/LConn1
  Current Sensor/RConn1 -- PS-Simulink Converter1/LConn1
  Current Sensor1/RConn2 -- Battery (Table-Based)/LConn1
  Voltage Sensor1/RConn1 -- PS-Simulink Converter2/LConn1
  Current Sensor1/RConn1 -- PS-Simulink Converter4/LConn1
  Battery (Table-Based)/LConn2 -- PS-Simulink Converter3/LConn1

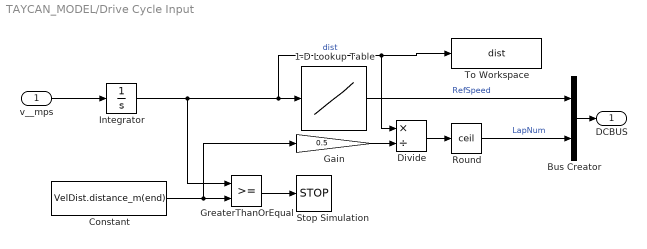
== system TAYCAN_MODEL/Drive Cycle Input ==
  v__mps : Inport
  1-D Lookup Table : Lookup_n-D  NumberOfTableDimensions=1  BreakpointsForDimension1=VelDist.distance_m  Table=VelDist.velocity_mps  InternalRulePriority=Speed  RndMeth=Simplest
  Bus Creator : BusCreator  Inputs=2
  Constant : Constant  Value=VelDist.distance_m(end)
  Divide : Product  Inputs=*/
  Gain : Gain  Gain=0.5
  GreaterThanOrEqual : RelationalOperator  OutDataTypeStr=boolean  RndMeth=Simplest  InputSameDT=off
  Integrator : Integrator
  Round : Rounding  Operator=ceil
  Stop Simulation : Stop
  To Workspace : ToWorkspace  VariableName=dist  SaveFormat=Timeseries  SampleTime=-1
  DCBUS : Outport
  wires:
  Round/1 -> Bus Creator/2  "LapNum"
  Bus Creator/1 -> DCBUS/1
  1-D Lookup Table/1 -> Bus Creator/1  "RefSpeed"
  v__mps/1 -> Integrator/1
  Integrator/1 -> To Workspace/1, Divide/1, 1-D Lookup Table/1, GreaterThanOrEqual/1  "dist"
  Constant/1 -> Gain/1, GreaterThanOrEqual/2
  Gain/1 -> Divide/2
  Divide/1 -> Round/1
  GreaterThanOrEqual/1 -> Stop Simulation/1

== system TAYCAN_MODEL/Driver ==
  DCBUS : Inport
  v__mps : Inport  Port=2
  Bus Creator : BusCreator  Inputs=3
  Bus Selector : BusSelector  OutputSignals=RefSpeed
  Longitudinal Driver1 : autolibshared/Longitudinal Driver  extAccelOvr=off  extDecelOvr=off  extAccelHld=off  extDecelHld=off  extAccelZero=off  extDecelZero=off  cntrlType=Predictive  shftType=None  velUnits=m/s  gearOut=off  Kp=Driver_Kp  Ki=Driver_Ki  Kff=Driver_Kff  Kg=Driver_Kg  VehVelVec=[0 100]  KffVec=[.1 .1]  KpVec=[10 10]  KiVec=[5 5]  KgVec=[0 0]  m=Tot_vehicle_mass_kg  Kpt=Kpt  tau=tau  L=L  aR=aR  bR=bR  cR=cR  g=g  vnom=100  Kaw=Driver_Kaw  tauerr=.03  tauPt=2  GearInit=0  tShift=.1  pdlVec=[0.1 0.4 0.5 0.9]  upShftTbl=[-1 12.9375 26.4375 39.9375 51.18749999999999 62.4375 72.84375 83.25;-1 16.3125 29.8125 43.3125 54.5624 65.8125 76.78125 87.75;-1 19.6875 33.1875 46.68749999999999 57.9375 69.1875 80.71875 92.25;-1 33 52.5 77.25 100.5 138.75 161.875 185]  dwnShftTbl=[1 9.5625 23.0625 36.5625 47.8125 59.0625 68.90625 78.75;1 12.9375 26.4375 39.9375 51.18749999999999 62.4375 72.84375 83.25;1 16.3125 29.8125 43.3125 54.562499 65.8125 76.78125 87.75;1 19.6875 33.1875 46.68749999999999 57.9375 69.1875 80.71875 92.25]  tClutch=.5  tRev=.5  tPark=120  aMode=1  UpGearVec="[0  1  2  3  4  5  6  7]"  DownGearVec="[1  2  3  4  5  6  7  8]"
  DBUS : Outport
  wires:
  DCBUS/1 -> Bus Selector/1
  v__mps/1 -> Longitudinal Driver1/2
  Longitudinal Driver1/1 -> Bus Creator/1  "Info"
  Bus Creator/1 -> DBUS/1
  Bus Selector/1 -> Longitudinal Driver1/1  "<RefSpeed>"
  Longitudinal Driver1/2 -> Bus Creator/2  "Accel"
  Longitudinal Driver1/3 -> Bus Creator/3  "Decel"

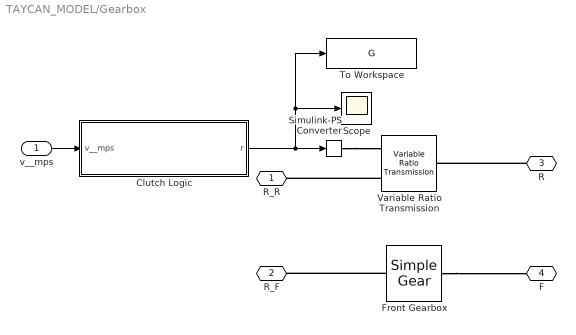
== system TAYCAN_MODEL/Gearbox ==
  v__mps : Inport
  Clutch Logic : Subsystem
  Front Gearbox : sdl_lib/Gears/Simple Gear  ratio=GFront  rotation_direction=sdl.enum.shaftOutputDirection.same  friction_model=sdl.enum.gear_efficiencies_load.off  T_noload=0.1 N*m  T_nom=5 N*m  efficiency_nom=0.8  efficiency=0.8  temperature_TLU=[280, 300, 320] K  load_TLU=[1, 5, 10] N*m  efficiency_TLU=[.95, .9, .85]  efficiency_TLU2=[.85, .8, .75; .95, .9, .85; .85, .8, .7]  w_thr=0.01 rad/s  pwr_thr=0.001 W  enable_backlash=false  hardstop_model=simscape.enum.hardstop.smooth  backlash_distance=1e-3 mm  r_base=0.1 m  transition=1e-4 mm  backlash_stiffness=1e6 N/m  backlash_damping=1e3 N*s/m  coeff_rest=0.7  v_tol=0.001 m/s  f_tol=0.001 N  mu_visc=[0, 0] N*m*s/rad  thermal_mass=50 J/K  temperature_specify=off  temperature_priority=High  temperature=300 K  temperature_nominal_specify=off  temperature_nominal_value=1  temperature_nominal_unit=K  x_backlash_specify=off  x_backlash_priority=None  x_backlash=0 mm  x_backlash_nominal_specify=off  x_backlash_nominal_value=1  x_backlash_nominal_unit=mm  f_hardstop_specify=off  f_hardstop_priority=None  f_hardstop=0 N  f_hardstop_nominal_specify=off  f_hardstop_nominal_value=1  f_hardstop_nominal_unit=N  v_backlash_specify=off  v_backlash_priority=None  v_backlash=0 m/s  v_backlash_nominal_specify=off  v_backlash_nominal_value=1  v_backlash_nominal_unit=m/s
  Scope : Scope
      settings: ActiveDisplayYMinimum=7.125  ActiveDisplayYMaximum=15.875  DataLoggingVariableName=ScopeData12
  Simulink-PS Converter : nesl_utility/Simulink-PS Converter  PhysicalDomain=network_engine_domain  SubClassName=ps_input  LeftPortType=input  RightPortType=output  PseudoPeriodic=off  Frequencies=[]  NoiseDistribution=none  NoiseParameters=[]  Unit=1  AffineConversion=off  FilteringAndDerivatives=provide  SimscapeFilterOrder=1  InputFilterTimeConstant=0.001  UdotUserProvided=0
  To Workspace : ToWorkspace  VariableName=G  SaveFormat=Timeseries  SampleTime=-1
  Variable Ratio Transmission : sdl_lib/Couplings & Drives/Variable Ratio Transmission  rotation_direction=sdl.enum.shaftOutputDirection.same  kp=5e5 N*m/rad  kv=5e3 N*m*s/rad  initial_torque=0 N*m  ratio_thr=0.01  losses_model=sdl.enum.lossesOffOn.off  efficiency=0.8  pwr_thr=0.001 W  mu_visc=[0, 0] N*m*s/rad
      settings: InternalSimscapePortConfiguration="{\"Bottom\":[],\"Left\":[{\"id\":\"ratio\",\"label\":\"r\",\"type\":\"input\"},{\"id\":\"B\",\"label\":\"B\",\"type\":\"foundation.mechanical.rotational.rotational\"}],\"Right\":[{\"id\":\"F\",\"label\":\"F\",\"type\":\"foundation.mechanical.rotational.rotational\"}],\"Top\":[]}"
  R_R : PMIOPort  Side=Left
  R_F : PMIOPort  Port=2  Side=Left
  R : PMIOPort  Port=3  Side=Right
  F : PMIOPort  Port=4  Side=Right
  wires:
  v__mps/1 -> Clutch Logic/1(v__mps)
  Clutch Logic/1(r) -> To Workspace/1, Scope/1, Simulink-PS Converter/1
  connections:
  Front Gearbox/LConn1 -- R_F/RConn1
  Front Gearbox/RConn1 -- F/RConn1
  R/RConn1 -- Variable Ratio Transmission/RConn1
  Variable Ratio Transmission/LConn2 -- R_R/RConn1
  Simulink-PS Converter/RConn1 -- Variable Ratio Transmission/LConn1

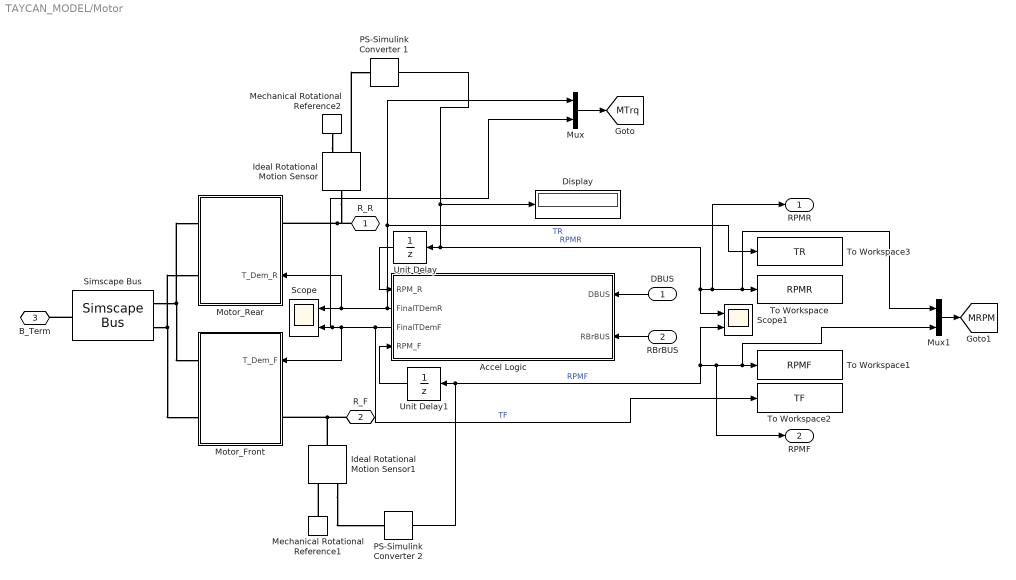
== system TAYCAN_MODEL/Motor ==
  DBUS : Inport
  RBrBUS : Inport  Port=2
  Accel Logic : Subsystem
      settings: PortSchema="{\"entries\":[{\"content\":{\"sides\":[{\"content\":{\"connectorIds\":[\"In1\",\"Out1\",\"Out2\",\"In2\"]},\"type\":\"ConnectorPlacement.EquallySpacedRectSide\",\"uuid\":\"baff776e-a3d5-4b10-b36e-e402d48273e8\"},{\"content\":{\"connectorIds\":[\"In3\",\"In4\"],\"side\":\"RIGHT\"},\"type\":\"ConnectorPlacement.EquallySpacedRectSide\",\"uuid\":\"49beed22-fcef-4cb3-b069-2a97db70d1f2\"},{\"content\":{\"side\":\"TOP\"},\"type\":\"ConnectorPlacement.EquallySpacedRectSide\",\"uuid\":\"b87adc78-e200-4142-97e4-24303affe0d6\"},{\"content\":{\"side\":\"BOTTOM\"},\"type\":\"ConnectorPlacement.EquallySpacedRectSide\",\"uuid\":\"18465ca1-6246-423f-acfb-1cf1616e3de5\"}]},\"type\":\"ConnectorPlacement.EquallySpacedConnector\",\"uuid\":\"977ce04e-c15c-41d4-8c59-6e70d5e20e05\"}],\"packageUris\":[\"http://schema.mathworks.com/mf0/Connector/R2020b\"],\"version\":\"1.0\"}"
  Display : Display
  Ideal Rotational Motion Sensor : fl_lib/Mechanical/Mechanical Sensors/Ideal Rotational Motion Sensor  reference=foundation.enum.MeasurementReference.difference  acceleration_port=false  velocity_port=true  position_port=false  wrap_angle=simscape.enum.onoff.off  offset=0 rad
      settings: InternalSimscapePortConfiguration="{\"Bottom\":[],\"Left\":[{\"id\":\"R\",\"label\":\"R\",\"type\":\"foundation.mechanical.rotational.rotational\"}],\"Right\":[{\"id\":\"C\",\"label\":\"C\",\"type\":\"foundation.mechanical.rotational.rotational\"},{\"id\":\"W\",\"label\":\"W\",\"type\":\"output\"}],\"Top\":[]}"
  Ideal Rotational Motion Sensor1 : fl_lib/Mechanical/Mechanical Sensors/Ideal Rotational Motion Sensor  reference=foundation.enum.MeasurementReference.difference  acceleration_port=false  velocity_port=true  position_port=false  wrap_angle=simscape.enum.onoff.off  offset=0 rad
      settings: InternalSimscapePortConfiguration="{\"Bottom\":[],\"Left\":[{\"id\":\"R\",\"label\":\"R\",\"type\":\"foundation.mechanical.rotational.rotational\"}],\"Right\":[{\"id\":\"C\",\"label\":\"C\",\"type\":\"foundation.mechanical.rotational.rotational\"},{\"id\":\"W\",\"label\":\"W\",\"type\":\"output\"}],\"Top\":[]}"
  Mechanical Rotational Reference1 : fl_lib/Mechanical/Rotational Elements/Mechanical Rotational Reference
  Mechanical Rotational Reference2 : fl_lib/Mechanical/Rotational Elements/Mechanical Rotational Reference
  Motor_Front : Subsystem
      settings: PortSchema="{\"entries\":[{\"content\":{\"sides\":[{\"content\":{\"connectorIds\":[\"LConn1\",\"LConn2\"]},\"type\":\"ConnectorPlacement.EquallySpacedRectSide\",\"uuid\":\"b2cd9267-5af1-4877-8b10-4fb12093f068\"},{\"content\":{\"connectorIds\":[\"In1\",\"RConn1\"],\"side\":\"RIGHT\"},\"type\":\"ConnectorPlacement.EquallySpacedRectSide\",\"uuid\":\"d3fd2355-7ec5-4b07-9d7b-20c5f535c0d0\"},{\"content\":{\"side\":\"TOP\"},\"type\":\"ConnectorPlacement.EquallySpacedRectSide\",\"uuid\":\"193d00b4-0d2c-45f8-a19c-63f28386a73a\"}]},\"type\":\"ConnectorPlacement.EquallySpacedConnector\",\"uuid\":\"b0a8a7c6-acc6-432b-88c8-22ff0c1fc1ab\"}],\"packageUris\":[\"http://schema.mathworks.com/mf0/Connector/R2020b\"],\"version\":\"1.0\"}"
  Motor_Rear : Subsystem
      settings: PortSchema="{\"entries\":[{\"content\":{\"sides\":[{\"content\":{\"connectorIds\":[\"LConn1\",\"LConn2\"]},\"type\":\"ConnectorPlacement.EquallySpacedRectSide\",\"uuid\":\"a4f09563-c033-4f6d-843e-a12dae0900e6\"},{\"content\":{\"connectorIds\":[\"RConn1\",\"In1\"],\"side\":\"RIGHT\"},\"type\":\"ConnectorPlacement.EquallySpacedRectSide\",\"uuid\":\"a4a49373-8430-4e89-8218-3611af14483f\"},{\"content\":{\"side\":\"TOP\"},\"type\":\"ConnectorPlacement.EquallySpacedRectSide\",\"uuid\":\"0cbad38e-68db-4d1d-b6fa-f6d8df1a71ec\"}]},\"type\":\"ConnectorPlacement.EquallySpacedConnector\",\"uuid\":\"b28fe165-9041-474c-84ec-c3e222dae80f\"}],\"packageUris\":[\"http://schema.mathworks.com/mf0/Connector/R2020b\"],\"version\":\"1.0\"}"
  Mux : Mux  Inputs=2
  Mux1 : Mux  Inputs=2
  PS-Simulink Converter 1 : nesl_utility/PS-Simulink Converter  PhysicalDomain=network_engine_domain  SubClassName=ps_output  LeftPortType=input  RightPortType=output  PseudoPeriodic=off  Frequencies=[]  VectorFormat=1-D array  Unit=rpm  AffineConversion=off
  PS-Simulink Converter 2 : nesl_utility/PS-Simulink Converter  PhysicalDomain=network_engine_domain  SubClassName=ps_output  LeftPortType=input  RightPortType=output  PseudoPeriodic=off  Frequencies=[]  VectorFormat=1-D array  Unit=rpm  AffineConversion=off
  Scope : Scope  NumInputPorts=2
      settings: ActiveDisplayYMinimum=-506.25  ActiveDisplayYMaximum=1056.25  DataLoggingVariableName=ScopeData5
  Scope1 : Scope  NumInputPorts=2
      settings: ActiveDisplayYMinimum=-1831.3871662583549  ActiveDisplayYMaximum=16482.4844963252  DataLoggingVariableName=ScopeData10
  Simscape Bus : SimscapeBus  HierarchyStrings=Pos;Neg
  To Workspace : ToWorkspace  VariableName=RPMR  SaveFormat=Timeseries  SampleTime=-1
  To Workspace1 : ToWorkspace  VariableName=RPMF  SaveFormat=Timeseries  SampleTime=-1
  To Workspace2 : ToWorkspace  VariableName=TF  SaveFormat=Timeseries  SampleTime=-1
  To Workspace3 : ToWorkspace  VariableName=TR  SaveFormat=Timeseries  SampleTime=-1
  Unit Delay : UnitDelay  SampleTime=-1  HasFrameUpgradeWarning=on
  Unit Delay1 : UnitDelay  SampleTime=-1  HasFrameUpgradeWarning=on
  R_R : PMIOPort  Side=Right
  R_F : PMIOPort  Port=2  Side=Right
  B_Term : PMIOPort  Port=3  Side=Right
  RPMR : Outport
  RPMF : Outport  Port=2
  tag scope: MRPM=global, MTrq=global
  wires:
  DBUS/1 -> Accel Logic/3(DBUS)
  RBrBUS/1 -> Accel Logic/4(RBrBUS)
  Accel Logic/1(FinalTDemR) -> Mux/1, To Workspace3/1, Motor_Rear/1(T_Dem_R), Scope/1  "TR"
  Accel Logic/2(FinalTDemF) -> Mux/2, Scope/2, Motor_Front/1(T_Dem_F), To Workspace2/1  "TF"
  PS-Simulink Converter 2/1 -> Scope1/2, RPMF/1, Mux1/2, To Workspace1/1, Unit Delay1/1  "RPMF"
  Unit Delay1/1 -> Accel Logic/2(RPM_F)
  Unit Delay/1 -> Accel Logic/1(RPM_R)
  PS-Simulink Converter 1/1 -> Display/1, Mux1/1, To Workspace/1, RPMR/1, Scope1/1, Unit Delay/1  "RPMR"
  Mux/1 -> [MTrq]
  Mux1/1 -> [MRPM]
  connections:
  Simscape Bus/RConn1 -- B_Term/RConn1
  Simscape Bus/LConn1 -- Motor_Front/LConn1 -- Motor_Rear/LConn1
  Simscape Bus/LConn2 -- Motor_Front/LConn2 -- Motor_Rear/LConn2
  R_R/RConn1 -- Ideal Rotational Motion Sensor/LConn1 -- Motor_Rear/RConn1
  R_F/RConn1 -- Ideal Rotational Motion Sensor1/LConn1 -- Motor_Front/RConn1
  Mechanical Rotational Reference2/LConn1 -- Ideal Rotational Motion Sensor/RConn1
  Ideal Rotational Motion Sensor/RConn2 -- PS-Simulink Converter 1/LConn1
  Mechanical Rotational Reference1/LConn1 -- Ideal Rotational Motion Sensor1/RConn1
  Ideal Rotational Motion Sensor1/RConn2 -- PS-Simulink Converter 2/LConn1
